simulink model "SIL_Autopilot_Vasarhelyi"  (R2020b)
settings: Solver=FixedStepAuto  StartTime=0  StopTime=T  FixedStep=0.01  RelTol=1e-3  EnableMultiTasking=on
model workspace (MAT data in the model file):
  SL_ROS_VariableLengthArrays_MaxSizes : object (value not decoded)
undefined symbols (not defined in the file): Altitude_ref, DiscIntNeverNeededParam, Elevators, p_swarm, Propeller, RightAileron, RightFlap, Rudder
libraries: robotlib x20, simulink x15
(part 2 of 5)

== system SIL_Autopilot_Vasarhelyi/Cessna 4/Attitude Control ==
  note: bota po
  Vel ref : Inport
  Euler Angles : Inport  Port=2
  Roll_ref : Inport  Port=3
  Altitude : Inport  Port=4
  Vel_in : Inport  Port=5
  Altitude ref : Inport  Port=6
  Bus Selector : BusSelector  OutputSignals=Pitch,Roll,Yaw
  Constant : Constant  Value=0
  Controle de Altitude : Subsystem
  Controle de Velocidade : Subsystem
  Gain : Gain  Gain=-1
  Servo : Subsystem
  Sum1 : Sum  Inputs=|+-
  Sum3 : Sum  Inputs=+-|
  Sum5 : Sum  Inputs=+-|
  Z Take-off Ref : Constant  Value=5
  Profundor : Outport
  Rudder : Outport  Port=2
  Aileron : Outport  Port=3
  Throtlle : Outport  Port=4
  altitude_e : Outport  Port=5
  velocity_e : Outport  Port=6
  roll_e : Outport  Port=7
  wires:
  Roll_ref/1 -> Sum1/1  "Roll Ref"
  Constant/1 -> Sum5/1  "Yaw Ref"
  Servo/4(Throtlle) -> Throtlle/1
  Servo/2(Aileron) -> Aileron/1
  Servo/3(Rudder) -> Rudder/1
  Servo/1(Profundor) -> Profundor/1
  Z Take-off Ref/1 -> Servo/6(Altitude Ref)
  Altitude/1 -> Controle de Altitude/2(Altitude), Servo/5(Altitude)
  Gain/1 -> Sum3/2
  Sum5/1 -> Servo/3(Yaw Attitude)
  Bus Selector/3 -> Sum5/2  "<Yaw>"
  Sum3/1 -> Servo/1(Pitch Attitude)
  Euler Angles/1 -> Bus Selector/1
  Bus Selector/1 -> Gain/1  "<Pitch>"
  Bus Selector/2 -> Sum1/2  "<Roll>"
  Controle de Velocidade/1(Propeller Target) -> Servo/4(Vel_in)
  Controle de Altitude/1(Pitch_ref) -> Sum3/1
  Vel ref/1 -> Controle de Velocidade/1(Velocity Ref)
  Altitude ref/1 -> Controle de Altitude/1(Altitude Ref)
  Sum1/1 -> roll_e/1, Servo/2(Roll Attitude)
  Vel_in/1 -> Controle de Velocidade/2(Velocity)
  Controle de Altitude/2(altitude_error) -> altitude_e/1
  Controle de Velocidade/2(velocity_error) -> velocity_e/1

== system SIL_Autopilot_Vasarhelyi/Cessna 4/Controle de Direção ==
  Yaw : Inport
  X : Inport  Port=2
  Y : Inport  Port=3
  Y Ref : Inport  Port=4
  X Ref : Inport  Port=5
  Atan2 : Trigonometry  Operator=atan2
  Discrete Derivative : simulink/Discrete/Discrete Derivative  gainval=1.0  ICPrevScaledInput=0.0  OutMin=[]  OutMax=[]  OutDataType=fixdt(1, 16)  OutScaling=2^-10  DoSatur=off
  Discrete-Time Integrator : DiscreteIntegrator  SampleTime=-1  ICPrevOutput=DiscIntNeverNeededParam  ICPrevScaledInput=DiscIntNeverNeededParam
  Kd : Gain  Gain=3.0
  Ki : Gain  Gain=0.0
  Kp : Gain  Gain=1.6616
  Mux1 : Mux  Inputs=2
  Mux2 : Mux  Inputs=2
  Mux3 : Mux  Inputs=2
  Saturation : Saturate  UpperLimit=0.226893  LowerLimit=-0.226893
  Sum2 : Sum  Inputs=|+-
  Sum3 : Sum  Inputs=|+-
  Sum4 : Sum  Inputs=|+-
  Sum5 : Sum  Inputs=+++
  neg : Gain  Gain=-1
  yaw_error : Outport
  Roll Ref : Outport  Port=2
  guidance_error : Outport  Port=3
  wires:
  Mux1/1 -> Mux3/1
  Mux2/1 -> Mux3/2
  Saturation/1 -> neg/1
  neg/1 -> Roll Ref/1
  Sum3/1 -> Atan2/1
  Y/1 -> Sum3/2, Mux2/2
  Y Ref/1 -> Sum3/1, Mux2/1
  X Ref/1 -> Sum2/1, Mux1/1
  X/1 -> Sum2/2, Mux1/2
  Sum2/1 -> Atan2/2
  Atan2/1 -> Sum4/1
  Yaw/1 -> Sum4/2
  Mux3/1 -> guidance_error/1
  Sum5/1 -> Saturation/1
  Kp/1 -> Sum5/2
  Kd/1 -> Sum5/1
  Discrete Derivative/1 -> Kd/1
  Discrete-Time Integrator/1 -> Ki/1
  Sum4/1 -> Discrete-Time Integrator/1, Kp/1, Discrete Derivative/1, yaw_error/1
  Ki/1 -> Sum5/3

== system SIL_Autopilot_Vasarhelyi/Cessna 4/Local Flocking Algorithm ==
  Pos : Inport
  Altitude ref : Inport  Port=2
  Xi : Inport  Port=3
  Bus Selector2 : BusSelector  OutputSignals=X,Y,Altitude
  Discrete Derivative : simulink/Discrete/Discrete Derivative  gainval=1.0  ICPrevScaledInput=0.0  OutMin=[]  OutMax=[]  OutDataType=fixdt(1, 16)  OutScaling=2^-10  DoSatur=off
  Gerador de Waypoints : Subsystem
  Mux : Mux  Inputs=3
  Mux1 : Mux  Inputs=3
  Vasarhelyi Algorithm : Subsystem
  Velocity Direction : MATLAB Function  TreatAsAtomicUnit=on
  Z : Display
  Y Ref : Outport
  X Ref : Outport  Port=2
  vel : Outport  Port=3
  u_ref : Outport  Port=4
  Waypoints : Outport  Port=5
  wires:
  Mux1/1 -> Waypoints/1, Velocity Direction/2(wp)
  Velocity Direction/1(u_ref) -> u_ref/1, Vasarhelyi Algorithm/3(u_ref)
  Pos/1 -> Bus Selector2/1
  Altitude ref/1 -> Mux1/3
  Gerador de Waypoints/2(Y Ref) -> Mux1/2
  Gerador de Waypoints/1(X Ref) -> Mux1/1
  Bus Selector2/1 -> Gerador de Waypoints/1(X State), Mux/1  "<X>"
  Bus Selector2/2 -> Gerador de Waypoints/2(Y State), Mux/2  "<Y>"
  Bus Selector2/3 -> Mux/3  "<Altitude>"
  Mux/1 -> Discrete Derivative/1, Vasarhelyi Algorithm/1(pos_i), Velocity Direction/1(pos)
  Discrete Derivative/1 -> vel/1
  Xi/1 -> Vasarhelyi Algorithm/2(pqj)
  Vasarhelyi Algorithm/1(X) -> X Ref/1
  Vasarhelyi Algorithm/2(Y) -> Y Ref/1
  Vasarhelyi Algorithm/3(Z) -> Z/1

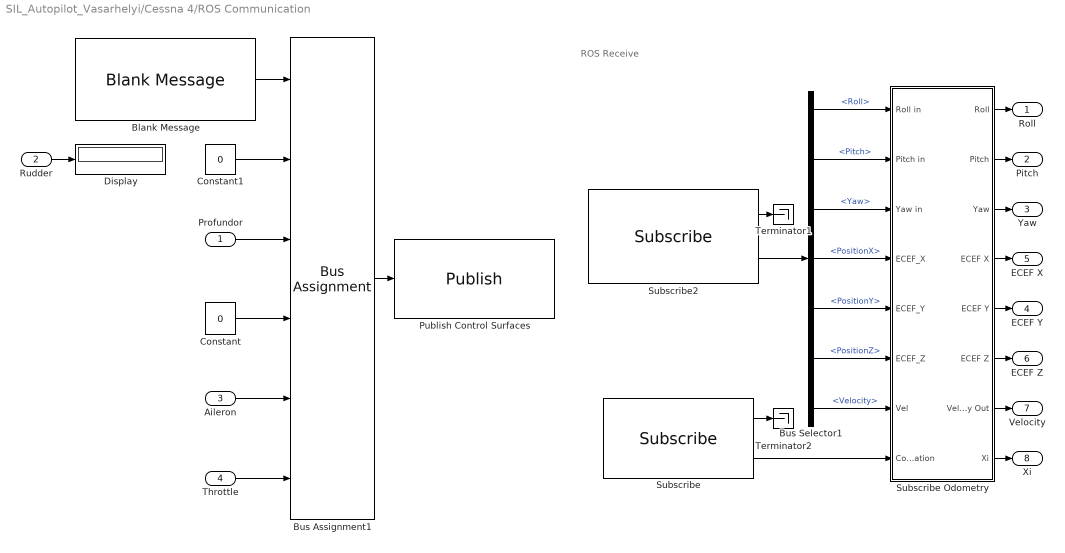
== system SIL_Autopilot_Vasarhelyi/Cessna 4/ROS Communication ==
  note: ROS Receive
  Profundor : Inport
  Rudder : Inport  Port=2
  Aileron : Inport  Port=3
  Throttle : Inport  Port=4
  Blank Message : robotlib/Blank Message  messageClass=Message  entityType=cessna_control/control_surfaces  messageType=cessna_control/control_surfaces  SampleTime=0.01  legacyBusStruct=off
  Bus Assignment1 : BusAssignment  AssignedSignals=Rudder,Elevators,RightFlap,RightAileron,Propeller
  Bus Selector1 : BusSelector  OutputSignals=Roll,Pitch,Yaw,PositionX,PositionY,PositionZ,Velocity
  Constant : Constant  Value=0
  Constant1 : Constant  Value=0
  Display : Display
  Publish Control Surfaces : robotlib/Publish  topicSource=Select from ROS network  topic=/uav4/cmd_control_surfaces  messageType=cessna_control/control_surfaces  legacyBusStruct=off  messageQueueLength=1
  Subscribe : robotlib/Subscribe  topicSource=Select from ROS network  topic=/uav4/Communication  messageType=aircraft_communication/NetworkComm  SampleTime=0.01  legacyBusStruct=off  messageQueueLength=1
  Subscribe Odometry : Subsystem  TreatAsAtomicUnit=on
  Subscribe2 : robotlib/Subscribe  topicSource=Select from ROS network  topic=/uav4/ground_truth/Odometry  messageType=aircraft_communication/Odom  SampleTime=0.01  legacyBusStruct=off  messageQueueLength=1
  Terminator1 : Terminator
  Terminator2 : Terminator
  Roll : Outport
  Pitch : Outport  Port=2
  Yaw : Outport  Port=3
  ECEF Y : Outport  Port=4
  ECEF X : Outport  Port=5
  ECEF Z : Outport  Port=6
  Velocity : Outport  Port=7
  Xi : Outport  Port=8
  wires:
  Profundor/1 -> Bus Assignment1/3
  Constant/1 -> Bus Assignment1/4
  Aileron/1 -> Bus Assignment1/5
  Subscribe Odometry/2(Pitch) -> Pitch/1
  Subscribe Odometry/4(ECEF X) -> ECEF X/1
  Subscribe Odometry/3(Yaw) -> Yaw/1
  Subscribe Odometry/1(Roll) -> Roll/1
  Subscribe Odometry/6(ECEF Z) -> ECEF Z/1
  Subscribe Odometry/7(Velocity Out) -> Velocity/1
  Rudder/1 -> Display/1
  Subscribe Odometry/8(Xi) -> Xi/1
  Throttle/1 -> Bus Assignment1/6
  Constant1/1 -> Bus Assignment1/2
  Bus Selector1/3 -> Subscribe Odometry/3(Yaw in)  "<Yaw>"
  Bus Assignment1/1 -> Publish Control Surfaces/1
  Bus Selector1/4 -> Subscribe Odometry/4(ECEF_X)  "<PositionX>"
  Bus Selector1/6 -> Subscribe Odometry/6(ECEF_Z)  "<PositionZ>"
  Blank Message/1 -> Bus Assignment1/1
  Subscribe/1 -> Terminator2/1
  Subscribe2/1 -> Terminator1/1
  Bus Selector1/2 -> Subscribe Odometry/2(Pitch in)  "<Pitch>"
  Subscribe/2 -> Subscribe Odometry/8(Communication)
  Bus Selector1/7 -> Subscribe Odometry/7(Vel)  "<Velocity>"
  Bus Selector1/1 -> Subscribe Odometry/1(Roll in)  "<Roll>"
  Bus Selector1/5 -> Subscribe Odometry/5(ECEF_Y)  "<PositionY>"
  Subscribe Odometry/5(ECEF Y) -> ECEF Y/1
  Subscribe2/2 -> Bus Selector1/1

== system SIL_Autopilot_Vasarhelyi/Cessna 5/Attitude Control ==
  note: bota po
  Vel ref : Inport
  Euler Angles : Inport  Port=2
  Roll_ref : Inport  Port=3
  Altitude : Inport  Port=4
  Vel_in : Inport  Port=5
  Altitude ref : Inport  Port=6
  Bus Selector : BusSelector  OutputSignals=Pitch,Roll,Yaw
  Constant : Constant  Value=0
  Controle de Altitude : Subsystem
  Controle de Velocidade : Subsystem
  Gain : Gain  Gain=-1
  Servo : Subsystem
  Sum1 : Sum  Inputs=|+-
  Sum3 : Sum  Inputs=+-|
  Sum5 : Sum  Inputs=+-|
  Z Take-off Ref : Constant  Value=5
  Profundor : Outport
  Rudder : Outport  Port=2
  Aileron : Outport  Port=3
  Throtlle : Outport  Port=4
  altitude_e : Outport  Port=5
  velocity_e : Outport  Port=6
  roll_e : Outport  Port=7
  wires:
  Roll_ref/1 -> Sum1/1  "Roll Ref"
  Constant/1 -> Sum5/1  "Yaw Ref"
  Servo/4(Throtlle) -> Throtlle/1
  Servo/2(Aileron) -> Aileron/1
  Servo/3(Rudder) -> Rudder/1
  Servo/1(Profundor) -> Profundor/1
  Z Take-off Ref/1 -> Servo/6(Altitude Ref)
  Altitude/1 -> Controle de Altitude/2(Altitude), Servo/5(Altitude)
  Gain/1 -> Sum3/2
  Sum5/1 -> Servo/3(Yaw Attitude)
  Bus Selector/3 -> Sum5/2  "<Yaw>"
  Sum3/1 -> Servo/1(Pitch Attitude)
  Euler Angles/1 -> Bus Selector/1
  Bus Selector/1 -> Gain/1  "<Pitch>"
  Bus Selector/2 -> Sum1/2  "<Roll>"
  Controle de Velocidade/1(Propeller Target) -> Servo/4(Vel_in)
  Controle de Altitude/1(Pitch_ref) -> Sum3/1
  Vel ref/1 -> Controle de Velocidade/1(Velocity Ref)
  Altitude ref/1 -> Controle de Altitude/1(Altitude Ref)
  Sum1/1 -> roll_e/1, Servo/2(Roll Attitude)
  Vel_in/1 -> Controle de Velocidade/2(Velocity)
  Controle de Altitude/2(altitude_error) -> altitude_e/1
  Controle de Velocidade/2(velocity_error) -> velocity_e/1

== system SIL_Autopilot_Vasarhelyi/Cessna 5/Controle de Direção ==
  Yaw : Inport
  X : Inport  Port=2
  Y : Inport  Port=3
  Y Ref : Inport  Port=4
  X Ref : Inport  Port=5
  Atan2 : Trigonometry  Operator=atan2
  Discrete Derivative : simulink/Discrete/Discrete Derivative  gainval=1.0  ICPrevScaledInput=0.0  OutMin=[]  OutMax=[]  OutDataType=fixdt(1, 16)  OutScaling=2^-10  DoSatur=off
  Discrete-Time Integrator : DiscreteIntegrator  SampleTime=-1  ICPrevOutput=DiscIntNeverNeededParam  ICPrevScaledInput=DiscIntNeverNeededParam
  Kd : Gain  Gain=3.0
  Ki : Gain  Gain=0.0
  Kp : Gain  Gain=1.6616
  Mux1 : Mux  Inputs=2
  Mux2 : Mux  Inputs=2
  Mux3 : Mux  Inputs=2
  Saturation : Saturate  UpperLimit=0.226893  LowerLimit=-0.226893
  Sum2 : Sum  Inputs=|+-
  Sum3 : Sum  Inputs=|+-
  Sum4 : Sum  Inputs=|+-
  Sum5 : Sum  Inputs=+++
  neg : Gain  Gain=-1
  yaw_error : Outport
  Roll Ref : Outport  Port=2
  guidance_error : Outport  Port=3
  wires:
  Mux1/1 -> Mux3/1
  Mux2/1 -> Mux3/2
  Saturation/1 -> neg/1
  neg/1 -> Roll Ref/1
  Sum3/1 -> Atan2/1
  Y/1 -> Sum3/2, Mux2/2
  Y Ref/1 -> Sum3/1, Mux2/1
  X Ref/1 -> Sum2/1, Mux1/1
  X/1 -> Sum2/2, Mux1/2
  Sum2/1 -> Atan2/2
  Atan2/1 -> Sum4/1
  Yaw/1 -> Sum4/2
  Mux3/1 -> guidance_error/1
  Sum5/1 -> Saturation/1
  Kp/1 -> Sum5/2
  Kd/1 -> Sum5/1
  Discrete Derivative/1 -> Kd/1
  Discrete-Time Integrator/1 -> Ki/1
  Sum4/1 -> Discrete-Time Integrator/1, Kp/1, Discrete Derivative/1, yaw_error/1
  Ki/1 -> Sum5/3

== system SIL_Autopilot_Vasarhelyi/Cessna 5/Local Flocking Algorithm ==
  Pos : Inport
  Altitude ref : Inport  Port=2
  Xi : Inport  Port=3
  Bus Selector2 : BusSelector  OutputSignals=X,Y,Altitude
  Discrete Derivative : simulink/Discrete/Discrete Derivative  gainval=1.0  ICPrevScaledInput=0.0  OutMin=[]  OutMax=[]  OutDataType=fixdt(1, 16)  OutScaling=2^-10  DoSatur=off
  Gerador de Waypoints : Subsystem
  Mux : Mux  Inputs=3
  Mux1 : Mux  Inputs=3
  Vasarhelyi Algorithm : Subsystem
  Velocity Direction : MATLAB Function  TreatAsAtomicUnit=on
  Z : Display
  Y Ref : Outport
  X Ref : Outport  Port=2
  vel : Outport  Port=3
  u_ref : Outport  Port=4
  Waypoints : Outport  Port=5
  wires:
  Mux1/1 -> Waypoints/1, Velocity Direction/2(wp)
  Velocity Direction/1(u_ref) -> u_ref/1, Vasarhelyi Algorithm/3(u_ref)
  Pos/1 -> Bus Selector2/1
  Altitude ref/1 -> Mux1/3
  Gerador de Waypoints/2(Y Ref) -> Mux1/2
  Gerador de Waypoints/1(X Ref) -> Mux1/1
  Bus Selector2/1 -> Gerador de Waypoints/1(X State), Mux/1  "<X>"
  Bus Selector2/2 -> Gerador de Waypoints/2(Y State), Mux/2  "<Y>"
  Bus Selector2/3 -> Mux/3  "<Altitude>"
  Mux/1 -> Discrete Derivative/1, Vasarhelyi Algorithm/1(pos_i), Velocity Direction/1(pos)
  Discrete Derivative/1 -> vel/1
  Xi/1 -> Vasarhelyi Algorithm/2(pqj)
  Vasarhelyi Algorithm/1(X) -> X Ref/1
  Vasarhelyi Algorithm/2(Y) -> Y Ref/1
  Vasarhelyi Algorithm/3(Z) -> Z/1

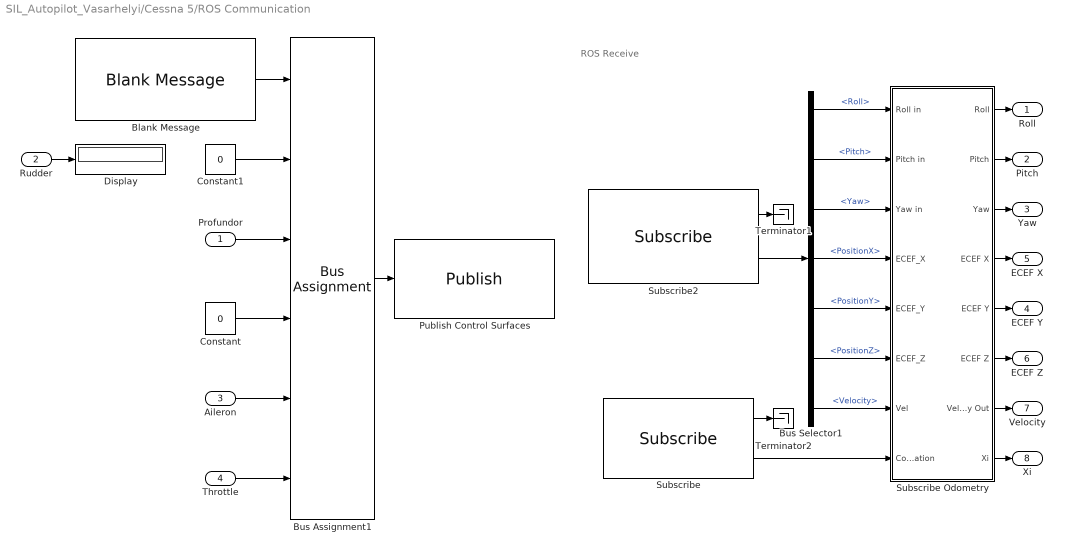
== system SIL_Autopilot_Vasarhelyi/Cessna 5/ROS Communication ==
  note: ROS Receive
  Profundor : Inport
  Rudder : Inport  Port=2
  Aileron : Inport  Port=3
  Throttle : Inport  Port=4
  Blank Message : robotlib/Blank Message  messageClass=Message  entityType=cessna_control/control_surfaces  messageType=cessna_control/control_surfaces  SampleTime=0.01  legacyBusStruct=off
  Bus Assignment1 : BusAssignment  AssignedSignals=Rudder,Elevators,RightFlap,RightAileron,Propeller
  Bus Selector1 : BusSelector  OutputSignals=Roll,Pitch,Yaw,PositionX,PositionY,PositionZ,Velocity
  Constant : Constant  Value=0
  Constant1 : Constant  Value=0
  Display : Display
  Publish Control Surfaces : robotlib/Publish  topicSource=Select from ROS network  topic=/uav5/cmd_control_surfaces  messageType=cessna_control/control_surfaces  legacyBusStruct=off  messageQueueLength=1
  Subscribe : robotlib/Subscribe  topicSource=Select from ROS network  topic=/uav5/Communication  messageType=aircraft_communication/NetworkComm  SampleTime=0.01  legacyBusStruct=off  messageQueueLength=1
  Subscribe Odometry : Subsystem  TreatAsAtomicUnit=on
  Subscribe2 : robotlib/Subscribe  topicSource=Select from ROS network  topic=/uav5/ground_truth/Odometry  messageType=aircraft_communication/Odom  SampleTime=0.01  legacyBusStruct=off  messageQueueLength=1
  Terminator1 : Terminator
  Terminator2 : Terminator
  Roll : Outport
  Pitch : Outport  Port=2
  Yaw : Outport  Port=3
  ECEF Y : Outport  Port=4
  ECEF X : Outport  Port=5
  ECEF Z : Outport  Port=6
  Velocity : Outport  Port=7
  Xi : Outport  Port=8
  wires:
  Profundor/1 -> Bus Assignment1/3
  Constant/1 -> Bus Assignment1/4
  Aileron/1 -> Bus Assignment1/5
  Subscribe Odometry/2(Pitch) -> Pitch/1
  Subscribe Odometry/4(ECEF X) -> ECEF X/1
  Subscribe Odometry/3(Yaw) -> Yaw/1
  Subscribe Odometry/1(Roll) -> Roll/1
  Subscribe Odometry/6(ECEF Z) -> ECEF Z/1
  Subscribe Odometry/7(Velocity Out) -> Velocity/1
  Rudder/1 -> Display/1
  Subscribe Odometry/8(Xi) -> Xi/1
  Throttle/1 -> Bus Assignment1/6
  Constant1/1 -> Bus Assignment1/2
  Bus Selector1/3 -> Subscribe Odometry/3(Yaw in)  "<Yaw>"
  Bus Assignment1/1 -> Publish Control Surfaces/1
  Bus Selector1/4 -> Subscribe Odometry/4(ECEF_X)  "<PositionX>"
  Bus Selector1/6 -> Subscribe Odometry/6(ECEF_Z)  "<PositionZ>"
  Blank Message/1 -> Bus Assignment1/1
  Subscribe/1 -> Terminator2/1
  Subscribe2/1 -> Terminator1/1
  Bus Selector1/2 -> Subscribe Odometry/2(Pitch in)  "<Pitch>"
  Subscribe/2 -> Subscribe Odometry/8(Communication)
  Bus Selector1/7 -> Subscribe Odometry/7(Vel)  "<Velocity>"
  Bus Selector1/1 -> Subscribe Odometry/1(Roll in)  "<Roll>"
  Bus Selector1/5 -> Subscribe Odometry/5(ECEF_Y)  "<PositionY>"
  Subscribe Odometry/5(ECEF Y) -> ECEF Y/1
  Subscribe2/2 -> Bus Selector1/1

== system SIL_Autopilot_Vasarhelyi/Cessna 1/Attitude Control/Controle de Altitude ==
  Altitude Ref : Inport
  Altitude : Inport  Port=2
  Derivative1 : Derivative
  Kd : Gain  Gain=0.00162
  Kp : Gain  Gain=0.1
  Saturation : Saturate  UpperLimit=0.785398  LowerLimit=-0.785398
  Sum : Sum  Inputs=|+-
  Sum5 : Sum  Inputs=++|
  Pitch_ref : Outport
  altitude_error : Outport  Port=2
  wires:
  Saturation/1 -> Pitch_ref/1
  Altitude Ref/1 -> Sum/1
  Altitude/1 -> Sum/2
  Kp/1 -> Sum5/2
  Kd/1 -> Sum5/1
  Derivative1/1 -> Kd/1
  Sum5/1 -> Saturation/1
  Sum/1 -> Derivative1/1, Kp/1, altitude_error/1

== system SIL_Autopilot_Vasarhelyi/Cessna 1/Attitude Control/Controle de Velocidade ==
  Velocity Ref : Inport
  Velocity : Inport  Port=2
  K_prop : Gain  Gain=0.08
  PID Velocidade : Subsystem
  Propeller Ref : Constant  Value=0.7
  Saturation3 : Saturate  UpperLimit=0.8  LowerLimit=0.6
  Sum1 : Sum  Inputs=+|+
  Sum7 : Sum  Inputs=+|-
  Target Propeller : Scope
  Velocity Error : Scope
  Propeller Target : Outport
  velocity_error : Outport  Port=2
  wires:
  Velocity/1 -> Sum7/2
  Velocity Ref/1 -> Sum7/1
  PID Velocidade/1(ev) -> K_prop/1
  Saturation3/1 -> Target Propeller/1, Propeller Target/1
  Propeller Ref/1 -> Sum1/2
  K_prop/1 -> Sum1/1
  Sum1/1 -> Saturation3/1
  Sum7/1 -> PID Velocidade/1(e_vel), velocity_error/1, Velocity Error/1

== system SIL_Autopilot_Vasarhelyi/Cessna 1/Attitude Control/Servo ==
  Pitch Attitude : Inport
  Roll Attitude : Inport  Port=2
  Yaw Attitude : Inport  Port=3
  Vel_in : Inport  Port=4
  Altitude : Inport  Port=5
  Altitude Ref : Inport  Port=6
  Gain1 : Gain  Gain=-1
  Gain2 : Gain
  Gain3 : Gain
  GreaterThanOrEqual : RelationalOperator  OutDataTypeStr=boolean  RndMeth=Simplest
  Saturation2 : Saturate  UpperLimit=0.0523599  LowerLimit=-0.0523599
  Saturation4 : Saturate  UpperLimit=0.0523599  LowerLimit=-0.0523599
  Saturation6 : Saturate  UpperLimit=0.0872665  LowerLimit=-0.0872665
  Switch{,1..3} (4 alike) : Switch  Criteria=u2 ~= 0
  Take-Off : Subsystem
  Profundor : Outport
  Aileron : Outport  Port=2
  Rudder : Outport  Port=3
  Throtlle : Outport  Port=4
  wires:
  GreaterThanOrEqual/1 -> Switch3/2, Switch2/2, Switch1/2, Switch/2
  Altitude Ref/1 -> GreaterThanOrEqual/2
  Take-Off/3(Rudder) -> Switch3/3
  Take-Off/2(Aileron) -> Switch2/3
  Altitude/1 -> GreaterThanOrEqual/1
  Switch3/1 -> Rudder/1
  Vel_in/1 -> Switch/1
  Switch/1 -> Throtlle/1
  Take-Off/4(Propeller) -> Switch/3
  Switch1/1 -> Profundor/1
  Take-Off/1(Elevators) -> Switch1/3
  Switch2/1 -> Aileron/1
  Saturation2/1 -> Switch2/1
  Saturation4/1 -> Switch1/1
  Saturation6/1 -> Switch3/1
  Gain1/1 -> Saturation6/1
  Yaw Attitude/1 -> Gain1/1
  Roll Attitude/1 -> Gain3/1
  Pitch Attitude/1 -> Gain2/1
  Gain2/1 -> Saturation4/1
  Gain3/1 -> Saturation2/1

== system SIL_Autopilot_Vasarhelyi/Cessna 1/Local Flocking Algorithm/Gerador de Waypoints ==
  X State : Inport
  Y State : Inport  Port=2
  Constant11 : Constant  Value=1000
  Constant13 : Constant  Value=-2000
  Constant14 : Constant  Value=-1000
  Constant5 : Constant  Value=-1000
  Constant6 : Constant  Value=1200
  Constant7 : Constant  Value=-1000
  Constant8 : Constant  Value=3000
  Constant9 : Constant  Value=-3000
  Demux : Demux  Outputs=8
  Display : Display
  Memory : Memory
  Próximo Waypoint : MATLAB Function  TreatAsAtomicUnit=on
  WayPoints : Mux  Inputs=8
  X Ref : Outport
  Y Ref : Outport  Port=2
  wires:
  Próximo Waypoint/2(Y_ref) -> Y Ref/1
  Próximo Waypoint/3(Estado) -> Display/1, Memory/1
  Próximo Waypoint/1(X_ref) -> X Ref/1
  Demux/1 -> Próximo Waypoint/1(wp1_X)
  Demux/2 -> Próximo Waypoint/2(wp1_Y)
  Demux/3 -> Próximo Waypoint/3(wp2_X)
  Demux/4 -> Próximo Waypoint/4(wp2_Y)
  Demux/5 -> Próximo Waypoint/5(wp3_X)
  Demux/6 -> Próximo Waypoint/6(wp3_Y)
  Demux/7 -> Próximo Waypoint/7(wp4_X)
  Demux/8 -> Próximo Waypoint/8(wp4_Y)
  WayPoints/1 -> Demux/1
  Y State/1 -> Próximo Waypoint/9(Y_med)
  X State/1 -> Próximo Waypoint/10(X_med)
  Constant7/1 -> WayPoints/2
  Constant6/1 -> WayPoints/1
  Constant9/1 -> WayPoints/4
  Constant8/1 -> WayPoints/3
  Constant5/1 -> WayPoints/5
  Constant11/1 -> WayPoints/6
  Constant14/1 -> WayPoints/8
  Constant13/1 -> WayPoints/7
  Memory/1 -> Próximo Waypoint/11("Estado ")

== system SIL_Autopilot_Vasarhelyi/Cessna 1/Local Flocking Algorithm/Vasarhelyi Algorithm ==
  pos_i : Inport
  pqj : Inport  Port=2
  u_ref : Inport  Port=3
  Agents Number : Constant  Value=5
  Demux : Demux  Outputs=3
  Discrete Derivative : simulink/Discrete/Discrete Derivative  gainval=1.0  ICPrevScaledInput=0.0  OutMin=[]  OutMax=[]  OutDataType=fixdt(1, 16)  OutScaling=2^-10  DoSatur=off
  Discrete-Time Integrator : DiscreteIntegrator  SampleTime=-1  ICPrevOutput=DiscIntNeverNeededParam  ICPrevScaledInput=DiscIntNeverNeededParam
  Parameters : Subsystem
  Vasarhelyi Algorithm : MATLAB Function  TreatAsAtomicUnit=on
  dt : Constant  Value=0.01
  pos and vel of uavs : MATLAB Function  TreatAsAtomicUnit=on
  r_agent : Constant  Value=15
  X : Outport
  Y : Outport  Port=2
  Z : Outport  Port=3
  wires:
  Agents Number/1 -> pos and vel of uavs/1(nb_agents)
  u_ref/1 -> Vasarhelyi Algorithm/4(u_ref)
  Vasarhelyi Algorithm/1(vel_command) -> Discrete-Time Integrator/1
  dt/1 -> Vasarhelyi Algorithm/5(dt)
  pqj/1 -> pos and vel of uavs/3(pqj)
  r_agent/1 -> Vasarhelyi Algorithm/6(r_agent)
  Discrete-Time Integrator/1 -> Demux/1
  pos and vel of uavs/1(pos) -> Vasarhelyi Algorithm/2(pos), Discrete Derivative/1
  Demux/2 -> Y/1
  pos_i/1 -> pos and vel of uavs/2(pos_i)
  Demux/1 -> X/1
  Demux/3 -> Z/1
  Discrete Derivative/1 -> Vasarhelyi Algorithm/3(vel)
  Parameters/1(p_swarm) -> Vasarhelyi Algorithm/1(p_swarm_par)

== system SIL_Autopilot_Vasarhelyi/Cessna 1/ROS Communication/Subscribe Odometry ==
  Roll in : Inport
  Pitch in : Inport  Port=2
  Yaw in : Inport  Port=3
  ECEF_X : Inport  Port=4
  ECEF_Y : Inport  Port=5
  ECEF_Z : Inport  Port=6
  Vel : Inport  Port=7
  Communication : Inport  Port=8
  Bus Selector3 : BusSelector  OutputSignals=Comms
  Roll : Outport
  Pitch : Outport  Port=2
  Yaw : Outport  Port=3
  ECEF X : Outport  Port=4
  ECEF Y : Outport  Port=5
  ECEF Z : Outport  Port=6
  Velocity Out : Outport  Port=7
  Xi : Outport  Port=8
  wires:
  Roll in/1 -> Roll/1
  Pitch in/1 -> Pitch/1
  Yaw in/1 -> Yaw/1
  Bus Selector3/1 -> Xi/1  "<Comms>"
  ECEF_Z/1 -> ECEF Z/1
  ECEF_Y/1 -> ECEF Y/1
  ECEF_X/1 -> ECEF X/1
  Communication/1 -> Bus Selector3/1
  Vel/1 -> Velocity Out/1

== system SIL_Autopilot_Vasarhelyi/Cessna 2/Attitude Control/Controle de Altitude ==
  Altitude Ref : Inport
  Altitude : Inport  Port=2
  Derivative1 : Derivative
  Kd : Gain  Gain=0.00162
  Kp : Gain  Gain=0.1
  Saturation : Saturate  UpperLimit=0.785398  LowerLimit=-0.785398
  Sum : Sum  Inputs=|+-
  Sum5 : Sum  Inputs=++|
  Pitch_ref : Outport
  altitude_error : Outport  Port=2
  wires:
  Saturation/1 -> Pitch_ref/1
  Altitude Ref/1 -> Sum/1
  Altitude/1 -> Sum/2
  Kp/1 -> Sum5/2
  Kd/1 -> Sum5/1
  Derivative1/1 -> Kd/1
  Sum5/1 -> Saturation/1
  Sum/1 -> Derivative1/1, Kp/1, altitude_error/1

== system SIL_Autopilot_Vasarhelyi/Cessna 2/Attitude Control/Controle de Velocidade ==
  Velocity Ref : Inport
  Velocity : Inport  Port=2
  K_prop : Gain  Gain=0.08
  PID Velocidade : Subsystem
  Propeller Ref : Constant  Value=0.7
  Saturation3 : Saturate  UpperLimit=0.8  LowerLimit=0.6
  Sum1 : Sum  Inputs=+|+
  Sum7 : Sum  Inputs=+|-
  Target Propeller : Scope
  Velocity Error : Scope
  Propeller Target : Outport
  velocity_error : Outport  Port=2
  wires:
  Velocity/1 -> Sum7/2
  Velocity Ref/1 -> Sum7/1
  PID Velocidade/1(ev) -> K_prop/1
  Saturation3/1 -> Target Propeller/1, Propeller Target/1
  Propeller Ref/1 -> Sum1/2
  K_prop/1 -> Sum1/1
  Sum1/1 -> Saturation3/1
  Sum7/1 -> PID Velocidade/1(e_vel), velocity_error/1, Velocity Error/1

== system SIL_Autopilot_Vasarhelyi/Cessna 2/Attitude Control/Servo ==
  Pitch Attitude : Inport
  Roll Attitude : Inport  Port=2
  Yaw Attitude : Inport  Port=3
  Vel_in : Inport  Port=4
  Altitude : Inport  Port=5
  Altitude Ref : Inport  Port=6
  Gain1 : Gain  Gain=-1
  Gain2 : Gain
  Gain3 : Gain
  GreaterThanOrEqual : RelationalOperator  OutDataTypeStr=boolean  RndMeth=Simplest
  Saturation2 : Saturate  UpperLimit=0.0523599  LowerLimit=-0.0523599
  Saturation4 : Saturate  UpperLimit=0.0523599  LowerLimit=-0.0523599
  Saturation6 : Saturate  UpperLimit=0.0872665  LowerLimit=-0.0872665
  Switch{,1..3} (4 alike) : Switch  Criteria=u2 ~= 0
  Take-Off : Subsystem
  Profundor : Outport
  Aileron : Outport  Port=2
  Rudder : Outport  Port=3
  Throtlle : Outport  Port=4
  wires:
  GreaterThanOrEqual/1 -> Switch3/2, Switch2/2, Switch1/2, Switch/2
  Altitude Ref/1 -> GreaterThanOrEqual/2
  Take-Off/3(Rudder) -> Switch3/3
  Take-Off/2(Aileron) -> Switch2/3
  Altitude/1 -> GreaterThanOrEqual/1
  Switch3/1 -> Rudder/1
  Vel_in/1 -> Switch/1
  Switch/1 -> Throtlle/1
  Take-Off/4(Propeller) -> Switch/3
  Switch1/1 -> Profundor/1
  Take-Off/1(Elevators) -> Switch1/3
  Switch2/1 -> Aileron/1
  Saturation2/1 -> Switch2/1
  Saturation4/1 -> Switch1/1
  Saturation6/1 -> Switch3/1
  Gain1/1 -> Saturation6/1
  Yaw Attitude/1 -> Gain1/1
  Roll Attitude/1 -> Gain3/1
  Pitch Attitude/1 -> Gain2/1
  Gain2/1 -> Saturation4/1
  Gain3/1 -> Saturation2/1

== system SIL_Autopilot_Vasarhelyi/Cessna 2/Local Flocking Algorithm/Gerador de Waypoints ==
  X State : Inport
  Y State : Inport  Port=2
  Constant11 : Constant  Value=1000
  Constant13 : Constant  Value=-2000
  Constant14 : Constant  Value=-1000
  Constant5 : Constant  Value=-1000
  Constant6 : Constant  Value=1200
  Constant7 : Constant  Value=-1000
  Constant8 : Constant  Value=3000
  Constant9 : Constant  Value=-3000
  Demux : Demux  Outputs=8
  Display : Display
  Memory : Memory
  Próximo Waypoint : MATLAB Function  TreatAsAtomicUnit=on
  WayPoints : Mux  Inputs=8
  X Ref : Outport
  Y Ref : Outport  Port=2
  wires:
  Próximo Waypoint/2(Y_ref) -> Y Ref/1
  Próximo Waypoint/3(Estado) -> Display/1, Memory/1
  Próximo Waypoint/1(X_ref) -> X Ref/1
  Demux/1 -> Próximo Waypoint/1(wp1_X)
  Demux/2 -> Próximo Waypoint/2(wp1_Y)
  Demux/3 -> Próximo Waypoint/3(wp2_X)
  Demux/4 -> Próximo Waypoint/4(wp2_Y)
  Demux/5 -> Próximo Waypoint/5(wp3_X)
  Demux/6 -> Próximo Waypoint/6(wp3_Y)
  Demux/7 -> Próximo Waypoint/7(wp4_X)
  Demux/8 -> Próximo Waypoint/8(wp4_Y)
  WayPoints/1 -> Demux/1
  Y State/1 -> Próximo Waypoint/9(Y_med)
  X State/1 -> Próximo Waypoint/10(X_med)
  Constant7/1 -> WayPoints/2
  Constant6/1 -> WayPoints/1
  Constant9/1 -> WayPoints/4
  Constant8/1 -> WayPoints/3
  Constant5/1 -> WayPoints/5
  Constant11/1 -> WayPoints/6
  Constant14/1 -> WayPoints/8
  Constant13/1 -> WayPoints/7
  Memory/1 -> Próximo Waypoint/11("Estado ")

== system SIL_Autopilot_Vasarhelyi/Cessna 2/Local Flocking Algorithm/Vasarhelyi Algorithm ==
  pos_i : Inport
  pqj : Inport  Port=2
  u_ref : Inport  Port=3
  Agents Number : Constant  Value=5
  Demux : Demux  Outputs=3
  Discrete Derivative : simulink/Discrete/Discrete Derivative  gainval=1.0  ICPrevScaledInput=0.0  OutMin=[]  OutMax=[]  OutDataType=fixdt(1, 16)  OutScaling=2^-10  DoSatur=off
  Discrete-Time Integrator : DiscreteIntegrator  SampleTime=-1  ICPrevOutput=DiscIntNeverNeededParam  ICPrevScaledInput=DiscIntNeverNeededParam
  Parameters : Subsystem
  Vasarhelyi Algorithm : MATLAB Function  TreatAsAtomicUnit=on
  dt : Constant  Value=0.01
  pos and vel of uavs : MATLAB Function  TreatAsAtomicUnit=on
  r_agent : Constant  Value=15
  X : Outport
  Y : Outport  Port=2
  Z : Outport  Port=3
  wires:
  Agents Number/1 -> pos and vel of uavs/1(nb_agents)
  u_ref/1 -> Vasarhelyi Algorithm/4(u_ref)
  Vasarhelyi Algorithm/1(vel_command) -> Discrete-Time Integrator/1
  dt/1 -> Vasarhelyi Algorithm/5(dt)
  pqj/1 -> pos and vel of uavs/3(pqj)
  r_agent/1 -> Vasarhelyi Algorithm/6(r_agent)
  Discrete-Time Integrator/1 -> Demux/1
  pos and vel of uavs/1(pos) -> Vasarhelyi Algorithm/2(pos), Discrete Derivative/1
  Demux/2 -> Y/1
  pos_i/1 -> pos and vel of uavs/2(pos_i)
  Demux/1 -> X/1
  Demux/3 -> Z/1
  Discrete Derivative/1 -> Vasarhelyi Algorithm/3(vel)
  Parameters/1(p_swarm) -> Vasarhelyi Algorithm/1(p_swarm_par)

== system SIL_Autopilot_Vasarhelyi/Cessna 2/ROS Communication/Subscribe Odometry ==
  Roll in : Inport
  Pitch in : Inport  Port=2
  Yaw in : Inport  Port=3
  ECEF_X : Inport  Port=4
  ECEF_Y : Inport  Port=5
  ECEF_Z : Inport  Port=6
  Vel : Inport  Port=7
  Communication : Inport  Port=8
  Bus Selector3 : BusSelector  OutputSignals=Comms
  Roll : Outport
  Pitch : Outport  Port=2
  Yaw : Outport  Port=3
  ECEF X : Outport  Port=4
  ECEF Y : Outport  Port=5
  ECEF Z : Outport  Port=6
  Velocity Out : Outport  Port=7
  Xi : Outport  Port=8
  wires:
  Roll in/1 -> Roll/1
  Pitch in/1 -> Pitch/1
  Yaw in/1 -> Yaw/1
  Bus Selector3/1 -> Xi/1  "<Comms>"
  ECEF_Z/1 -> ECEF Z/1
  ECEF_Y/1 -> ECEF Y/1
  ECEF_X/1 -> ECEF X/1
  Communication/1 -> Bus Selector3/1
  Vel/1 -> Velocity Out/1

== system SIL_Autopilot_Vasarhelyi/Cessna 3/Attitude Control/Controle de Altitude ==
  Altitude Ref : Inport
  Altitude : Inport  Port=2
  Derivative1 : Derivative
  Kd : Gain  Gain=0.00162
  Kp : Gain  Gain=0.1
  Saturation : Saturate  UpperLimit=0.785398  LowerLimit=-0.785398
  Sum : Sum  Inputs=|+-
  Sum5 : Sum  Inputs=++|
  Pitch_ref : Outport
  altitude_error : Outport  Port=2
  wires:
  Saturation/1 -> Pitch_ref/1
  Altitude Ref/1 -> Sum/1
  Altitude/1 -> Sum/2
  Kp/1 -> Sum5/2
  Kd/1 -> Sum5/1
  Derivative1/1 -> Kd/1
  Sum5/1 -> Saturation/1
  Sum/1 -> Derivative1/1, Kp/1, altitude_error/1

== system SIL_Autopilot_Vasarhelyi/Cessna 3/Attitude Control/Controle de Velocidade ==
  Velocity Ref : Inport
  Velocity : Inport  Port=2
  K_prop : Gain  Gain=0.08
  PID Velocidade : Subsystem
  Propeller Ref : Constant  Value=0.7
  Saturation3 : Saturate  UpperLimit=0.8  LowerLimit=0.6
  Sum1 : Sum  Inputs=+|+
  Sum7 : Sum  Inputs=+|-
  Target Propeller : Scope
  Velocity Error : Scope
  Propeller Target : Outport
  velocity_error : Outport  Port=2
  wires:
  Velocity/1 -> Sum7/2
  Velocity Ref/1 -> Sum7/1
  PID Velocidade/1(ev) -> K_prop/1
  Saturation3/1 -> Target Propeller/1, Propeller Target/1
  Propeller Ref/1 -> Sum1/2
  K_prop/1 -> Sum1/1
  Sum1/1 -> Saturation3/1
  Sum7/1 -> PID Velocidade/1(e_vel), velocity_error/1, Velocity Error/1

== system SIL_Autopilot_Vasarhelyi/Cessna 3/Attitude Control/Servo ==
  Pitch Attitude : Inport
  Roll Attitude : Inport  Port=2
  Yaw Attitude : Inport  Port=3
  Vel_in : Inport  Port=4
  Altitude : Inport  Port=5
  Altitude Ref : Inport  Port=6
  Gain1 : Gain  Gain=-1
  Gain2 : Gain
  Gain3 : Gain
  GreaterThanOrEqual : RelationalOperator  OutDataTypeStr=boolean  RndMeth=Simplest
  Saturation2 : Saturate  UpperLimit=0.0523599  LowerLimit=-0.0523599
  Saturation4 : Saturate  UpperLimit=0.0523599  LowerLimit=-0.0523599
  Saturation6 : Saturate  UpperLimit=0.0872665  LowerLimit=-0.0872665
  Switch{,1..3} (4 alike) : Switch  Criteria=u2 ~= 0
  Take-Off : Subsystem
  Profundor : Outport
  Aileron : Outport  Port=2
  Rudder : Outport  Port=3
  Throtlle : Outport  Port=4
  wires:
  GreaterThanOrEqual/1 -> Switch3/2, Switch2/2, Switch1/2, Switch/2
  Altitude Ref/1 -> GreaterThanOrEqual/2
  Take-Off/3(Rudder) -> Switch3/3
  Take-Off/2(Aileron) -> Switch2/3
  Altitude/1 -> GreaterThanOrEqual/1
  Switch3/1 -> Rudder/1
  Vel_in/1 -> Switch/1
  Switch/1 -> Throtlle/1
  Take-Off/4(Propeller) -> Switch/3
  Switch1/1 -> Profundor/1
  Take-Off/1(Elevators) -> Switch1/3
  Switch2/1 -> Aileron/1
  Saturation2/1 -> Switch2/1
  Saturation4/1 -> Switch1/1
  Saturation6/1 -> Switch3/1
  Gain1/1 -> Saturation6/1
  Yaw Attitude/1 -> Gain1/1
  Roll Attitude/1 -> Gain3/1
  Pitch Attitude/1 -> Gain2/1
  Gain2/1 -> Saturation4/1
  Gain3/1 -> Saturation2/1

== system SIL_Autopilot_Vasarhelyi/Cessna 3/Local Flocking Algorithm/Gerador de Waypoints ==
  X State : Inport
  Y State : Inport  Port=2
  Constant11 : Constant  Value=1000
  Constant13 : Constant  Value=-2000
  Constant14 : Constant  Value=-1000
  Constant5 : Constant  Value=-1000
  Constant6 : Constant  Value=1200
  Constant7 : Constant  Value=-1000
  Constant8 : Constant  Value=3000
  Constant9 : Constant  Value=-3000
  Demux : Demux  Outputs=8
  Display : Display
  Memory : Memory
  Próximo Waypoint : MATLAB Function  TreatAsAtomicUnit=on
  WayPoints : Mux  Inputs=8
  X Ref : Outport
  Y Ref : Outport  Port=2
  wires:
  Próximo Waypoint/2(Y_ref) -> Y Ref/1
  Próximo Waypoint/3(Estado) -> Display/1, Memory/1
  Próximo Waypoint/1(X_ref) -> X Ref/1
  Demux/1 -> Próximo Waypoint/1(wp1_X)
  Demux/2 -> Próximo Waypoint/2(wp1_Y)
  Demux/3 -> Próximo Waypoint/3(wp2_X)
  Demux/4 -> Próximo Waypoint/4(wp2_Y)
  Demux/5 -> Próximo Waypoint/5(wp3_X)
  Demux/6 -> Próximo Waypoint/6(wp3_Y)
  Demux/7 -> Próximo Waypoint/7(wp4_X)
  Demux/8 -> Próximo Waypoint/8(wp4_Y)
  WayPoints/1 -> Demux/1
  Y State/1 -> Próximo Waypoint/9(Y_med)
  X State/1 -> Próximo Waypoint/10(X_med)
  Constant7/1 -> WayPoints/2
  Constant6/1 -> WayPoints/1
  Constant9/1 -> WayPoints/4
  Constant8/1 -> WayPoints/3
  Constant5/1 -> WayPoints/5
  Constant11/1 -> WayPoints/6
  Constant14/1 -> WayPoints/8
  Constant13/1 -> WayPoints/7
  Memory/1 -> Próximo Waypoint/11("Estado ")

== system SIL_Autopilot_Vasarhelyi/Cessna 3/Local Flocking Algorithm/Vasarhelyi Algorithm ==
  pos_i : Inport
  pqj : Inport  Port=2
  u_ref : Inport  Port=3
  Agents Number : Constant  Value=5
  Demux : Demux  Outputs=3
  Discrete Derivative : simulink/Discrete/Discrete Derivative  gainval=1.0  ICPrevScaledInput=0.0  OutMin=[]  OutMax=[]  OutDataType=fixdt(1, 16)  OutScaling=2^-10  DoSatur=off
  Discrete-Time Integrator : DiscreteIntegrator  SampleTime=-1  ICPrevOutput=DiscIntNeverNeededParam  ICPrevScaledInput=DiscIntNeverNeededParam
  Parameters : Subsystem
  Vasarhelyi Algorithm : MATLAB Function  TreatAsAtomicUnit=on
  dt : Constant  Value=0.01
  pos and vel of uavs : MATLAB Function  TreatAsAtomicUnit=on
  r_agent : Constant  Value=15
  X : Outport
  Y : Outport  Port=2
  Z : Outport  Port=3
  wires:
  Agents Number/1 -> pos and vel of uavs/1(nb_agents)
  u_ref/1 -> Vasarhelyi Algorithm/4(u_ref)
  Vasarhelyi Algorithm/1(vel_command) -> Discrete-Time Integrator/1
  dt/1 -> Vasarhelyi Algorithm/5(dt)
  pqj/1 -> pos and vel of uavs/3(pqj)
  r_agent/1 -> Vasarhelyi Algorithm/6(r_agent)
  Discrete-Time Integrator/1 -> Demux/1
  pos and vel of uavs/1(pos) -> Vasarhelyi Algorithm/2(pos), Discrete Derivative/1
  Demux/2 -> Y/1
  pos_i/1 -> pos and vel of uavs/2(pos_i)
  Demux/1 -> X/1
  Demux/3 -> Z/1
  Discrete Derivative/1 -> Vasarhelyi Algorithm/3(vel)
  Parameters/1(p_swarm) -> Vasarhelyi Algorithm/1(p_swarm_par)

== system SIL_Autopilot_Vasarhelyi/Cessna 3/ROS Communication/Subscribe Odometry ==
  Roll in : Inport
  Pitch in : Inport  Port=2
  Yaw in : Inport  Port=3
  ECEF_X : Inport  Port=4
  ECEF_Y : Inport  Port=5
  ECEF_Z : Inport  Port=6
  Vel : Inport  Port=7
  Communication : Inport  Port=8
  Bus Selector3 : BusSelector  OutputSignals=Comms
  Roll : Outport
  Pitch : Outport  Port=2
  Yaw : Outport  Port=3
  ECEF X : Outport  Port=4
  ECEF Y : Outport  Port=5
  ECEF Z : Outport  Port=6
  Velocity Out : Outport  Port=7
  Xi : Outport  Port=8
  wires:
  Roll in/1 -> Roll/1
  Pitch in/1 -> Pitch/1
  Yaw in/1 -> Yaw/1
  Bus Selector3/1 -> Xi/1  "<Comms>"
  ECEF_Z/1 -> ECEF Z/1
  ECEF_Y/1 -> ECEF Y/1
  ECEF_X/1 -> ECEF X/1
  Communication/1 -> Bus Selector3/1
  Vel/1 -> Velocity Out/1

== system SIL_Autopilot_Vasarhelyi/Cessna 4/Attitude Control/Controle de Altitude ==
  Altitude Ref : Inport
  Altitude : Inport  Port=2
  Derivative1 : Derivative
  Kd : Gain  Gain=0.00162
  Kp : Gain  Gain=0.1
  Saturation : Saturate  UpperLimit=0.785398  LowerLimit=-0.785398
  Sum : Sum  Inputs=|+-
  Sum5 : Sum  Inputs=++|
  Pitch_ref : Outport
  altitude_error : Outport  Port=2
  wires:
  Saturation/1 -> Pitch_ref/1
  Altitude Ref/1 -> Sum/1
  Altitude/1 -> Sum/2
  Kp/1 -> Sum5/2
  Kd/1 -> Sum5/1
  Derivative1/1 -> Kd/1
  Sum5/1 -> Saturation/1
  Sum/1 -> Derivative1/1, Kp/1, altitude_error/1

== system SIL_Autopilot_Vasarhelyi/Cessna 4/Attitude Control/Controle de Velocidade ==
  Velocity Ref : Inport
  Velocity : Inport  Port=2
  K_prop : Gain  Gain=0.08
  PID Velocidade : Subsystem
  Propeller Ref : Constant  Value=0.7
  Saturation3 : Saturate  UpperLimit=0.8  LowerLimit=0.6
  Sum1 : Sum  Inputs=+|+
  Sum7 : Sum  Inputs=+|-
  Target Propeller : Scope
  Velocity Error : Scope
  Propeller Target : Outport
  velocity_error : Outport  Port=2
  wires:
  Velocity/1 -> Sum7/2
  Velocity Ref/1 -> Sum7/1
  PID Velocidade/1(ev) -> K_prop/1
  Saturation3/1 -> Target Propeller/1, Propeller Target/1
  Propeller Ref/1 -> Sum1/2
  K_prop/1 -> Sum1/1
  Sum1/1 -> Saturation3/1
  Sum7/1 -> PID Velocidade/1(e_vel), velocity_error/1, Velocity Error/1

== system SIL_Autopilot_Vasarhelyi/Cessna 4/Attitude Control/Servo ==
  Pitch Attitude : Inport
  Roll Attitude : Inport  Port=2
  Yaw Attitude : Inport  Port=3
  Vel_in : Inport  Port=4
  Altitude : Inport  Port=5
  Altitude Ref : Inport  Port=6
  Gain1 : Gain  Gain=-1
  Gain2 : Gain
  Gain3 : Gain
  GreaterThanOrEqual : RelationalOperator  OutDataTypeStr=boolean  RndMeth=Simplest
  Saturation2 : Saturate  UpperLimit=0.0523599  LowerLimit=-0.0523599
  Saturation4 : Saturate  UpperLimit=0.0523599  LowerLimit=-0.0523599
  Saturation6 : Saturate  UpperLimit=0.0872665  LowerLimit=-0.0872665
  Switch{,1..3} (4 alike) : Switch  Criteria=u2 ~= 0
  Take-Off : Subsystem
  Profundor : Outport
  Aileron : Outport  Port=2
  Rudder : Outport  Port=3
  Throtlle : Outport  Port=4
  wires:
  GreaterThanOrEqual/1 -> Switch3/2, Switch2/2, Switch1/2, Switch/2
  Altitude Ref/1 -> GreaterThanOrEqual/2
  Take-Off/3(Rudder) -> Switch3/3
  Take-Off/2(Aileron) -> Switch2/3
  Altitude/1 -> GreaterThanOrEqual/1
  Switch3/1 -> Rudder/1
  Vel_in/1 -> Switch/1
  Switch/1 -> Throtlle/1
  Take-Off/4(Propeller) -> Switch/3
  Switch1/1 -> Profundor/1
  Take-Off/1(Elevators) -> Switch1/3
  Switch2/1 -> Aileron/1
  Saturation2/1 -> Switch2/1
  Saturation4/1 -> Switch1/1
  Saturation6/1 -> Switch3/1
  Gain1/1 -> Saturation6/1
  Yaw Attitude/1 -> Gain1/1
  Roll Attitude/1 -> Gain3/1
  Pitch Attitude/1 -> Gain2/1
  Gain2/1 -> Saturation4/1
  Gain3/1 -> Saturation2/1

== system SIL_Autopilot_Vasarhelyi/Cessna 4/Local Flocking Algorithm/Gerador de Waypoints ==
  X State : Inport
  Y State : Inport  Port=2
  Constant11 : Constant  Value=1000
  Constant13 : Constant  Value=-2000
  Constant14 : Constant  Value=-1000
  Constant5 : Constant  Value=-1000
  Constant6 : Constant  Value=1200
  Constant7 : Constant  Value=-1000
  Constant8 : Constant  Value=3000
  Constant9 : Constant  Value=-3000
  Demux : Demux  Outputs=8
  Display : Display
  Memory : Memory
  Próximo Waypoint : MATLAB Function  TreatAsAtomicUnit=on
  WayPoints : Mux  Inputs=8
  X Ref : Outport
  Y Ref : Outport  Port=2
  wires:
  Próximo Waypoint/2(Y_ref) -> Y Ref/1
  Próximo Waypoint/3(Estado) -> Display/1, Memory/1
  Próximo Waypoint/1(X_ref) -> X Ref/1
  Demux/1 -> Próximo Waypoint/1(wp1_X)
  Demux/2 -> Próximo Waypoint/2(wp1_Y)
  Demux/3 -> Próximo Waypoint/3(wp2_X)
  Demux/4 -> Próximo Waypoint/4(wp2_Y)
  Demux/5 -> Próximo Waypoint/5(wp3_X)
  Demux/6 -> Próximo Waypoint/6(wp3_Y)
  Demux/7 -> Próximo Waypoint/7(wp4_X)
  Demux/8 -> Próximo Waypoint/8(wp4_Y)
  WayPoints/1 -> Demux/1
  Y State/1 -> Próximo Waypoint/9(Y_med)
  X State/1 -> Próximo Waypoint/10(X_med)
  Constant7/1 -> WayPoints/2
  Constant6/1 -> WayPoints/1
  Constant9/1 -> WayPoints/4
  Constant8/1 -> WayPoints/3
  Constant5/1 -> WayPoints/5
  Constant11/1 -> WayPoints/6
  Constant14/1 -> WayPoints/8
  Constant13/1 -> WayPoints/7
  Memory/1 -> Próximo Waypoint/11("Estado ")

== system SIL_Autopilot_Vasarhelyi/Cessna 4/Local Flocking Algorithm/Vasarhelyi Algorithm ==
  pos_i : Inport
  pqj : Inport  Port=2
  u_ref : Inport  Port=3
  Agents Number : Constant  Value=5
  Demux : Demux  Outputs=3
  Discrete Derivative : simulink/Discrete/Discrete Derivative  gainval=1.0  ICPrevScaledInput=0.0  OutMin=[]  OutMax=[]  OutDataType=fixdt(1, 16)  OutScaling=2^-10  DoSatur=off
  Discrete-Time Integrator : DiscreteIntegrator  SampleTime=-1  ICPrevOutput=DiscIntNeverNeededParam  ICPrevScaledInput=DiscIntNeverNeededParam
  Parameters : Subsystem
  Vasarhelyi Algorithm : MATLAB Function  TreatAsAtomicUnit=on
  dt : Constant  Value=0.01
  pos and vel of uavs : MATLAB Function  TreatAsAtomicUnit=on
  r_agent : Constant  Value=15
  X : Outport
  Y : Outport  Port=2
  Z : Outport  Port=3
  wires:
  Agents Number/1 -> pos and vel of uavs/1(nb_agents)
  u_ref/1 -> Vasarhelyi Algorithm/4(u_ref)
  Vasarhelyi Algorithm/1(vel_command) -> Discrete-Time Integrator/1
  dt/1 -> Vasarhelyi Algorithm/5(dt)
  pqj/1 -> pos and vel of uavs/3(pqj)
  r_agent/1 -> Vasarhelyi Algorithm/6(r_agent)
  Discrete-Time Integrator/1 -> Demux/1
  pos and vel of uavs/1(pos) -> Vasarhelyi Algorithm/2(pos), Discrete Derivative/1
  Demux/2 -> Y/1
  pos_i/1 -> pos and vel of uavs/2(pos_i)
  Demux/1 -> X/1
  Demux/3 -> Z/1
  Discrete Derivative/1 -> Vasarhelyi Algorithm/3(vel)
  Parameters/1(p_swarm) -> Vasarhelyi Algorithm/1(p_swarm_par)

== system SIL_Autopilot_Vasarhelyi/Cessna 4/ROS Communication/Subscribe Odometry ==
  Roll in : Inport
  Pitch in : Inport  Port=2
  Yaw in : Inport  Port=3
  ECEF_X : Inport  Port=4
  ECEF_Y : Inport  Port=5
  ECEF_Z : Inport  Port=6
  Vel : Inport  Port=7
  Communication : Inport  Port=8
  Bus Selector3 : BusSelector  OutputSignals=Comms
  Roll : Outport
  Pitch : Outport  Port=2
  Yaw : Outport  Port=3
  ECEF X : Outport  Port=4
  ECEF Y : Outport  Port=5
  ECEF Z : Outport  Port=6
  Velocity Out : Outport  Port=7
  Xi : Outport  Port=8
  wires:
  Roll in/1 -> Roll/1
  Pitch in/1 -> Pitch/1
  Yaw in/1 -> Yaw/1
  Bus Selector3/1 -> Xi/1  "<Comms>"
  ECEF_Z/1 -> ECEF Z/1
  ECEF_Y/1 -> ECEF Y/1
  ECEF_X/1 -> ECEF X/1
  Communication/1 -> Bus Selector3/1
  Vel/1 -> Velocity Out/1

== system SIL_Autopilot_Vasarhelyi/Cessna 5/Attitude Control/Controle de Altitude ==
  Altitude Ref : Inport
  Altitude : Inport  Port=2
  Derivative1 : Derivative
  Kd : Gain  Gain=0.00162
  Kp : Gain  Gain=0.1
  Saturation : Saturate  UpperLimit=0.785398  LowerLimit=-0.785398
  Sum : Sum  Inputs=|+-
  Sum5 : Sum  Inputs=++|
  Pitch_ref : Outport
  altitude_error : Outport  Port=2
  wires:
  Saturation/1 -> Pitch_ref/1
  Altitude Ref/1 -> Sum/1
  Altitude/1 -> Sum/2
  Kp/1 -> Sum5/2
  Kd/1 -> Sum5/1
  Derivative1/1 -> Kd/1
  Sum5/1 -> Saturation/1
  Sum/1 -> Derivative1/1, Kp/1, altitude_error/1

== system SIL_Autopilot_Vasarhelyi/Cessna 5/Attitude Control/Controle de Velocidade ==
  Velocity Ref : Inport
  Velocity : Inport  Port=2
  K_prop : Gain  Gain=0.08
  PID Velocidade : Subsystem
  Propeller Ref : Constant  Value=0.7
  Saturation3 : Saturate  UpperLimit=0.8  LowerLimit=0.6
  Sum1 : Sum  Inputs=+|+
  Sum7 : Sum  Inputs=+|-
  Target Propeller : Scope
  Velocity Error : Scope
  Propeller Target : Outport
  velocity_error : Outport  Port=2
  wires:
  Velocity/1 -> Sum7/2
  Velocity Ref/1 -> Sum7/1
  PID Velocidade/1(ev) -> K_prop/1
  Saturation3/1 -> Target Propeller/1, Propeller Target/1
  Propeller Ref/1 -> Sum1/2
  K_prop/1 -> Sum1/1
  Sum1/1 -> Saturation3/1
  Sum7/1 -> PID Velocidade/1(e_vel), velocity_error/1, Velocity Error/1

== system SIL_Autopilot_Vasarhelyi/Cessna 5/Attitude Control/Servo ==
  Pitch Attitude : Inport
  Roll Attitude : Inport  Port=2
  Yaw Attitude : Inport  Port=3
  Vel_in : Inport  Port=4
  Altitude : Inport  Port=5
  Altitude Ref : Inport  Port=6
  Gain1 : Gain  Gain=-1
  Gain2 : Gain
  Gain3 : Gain
  GreaterThanOrEqual : RelationalOperator  OutDataTypeStr=boolean  RndMeth=Simplest
  Saturation2 : Saturate  UpperLimit=0.0523599  LowerLimit=-0.0523599
  Saturation4 : Saturate  UpperLimit=0.0523599  LowerLimit=-0.0523599
  Saturation6 : Saturate  UpperLimit=0.0872665  LowerLimit=-0.0872665
  Switch{,1..3} (4 alike) : Switch  Criteria=u2 ~= 0
  Take-Off : Subsystem
  Profundor : Outport
  Aileron : Outport  Port=2
  Rudder : Outport  Port=3
  Throtlle : Outport  Port=4
  wires:
  GreaterThanOrEqual/1 -> Switch3/2, Switch2/2, Switch1/2, Switch/2
  Altitude Ref/1 -> GreaterThanOrEqual/2
  Take-Off/3(Rudder) -> Switch3/3
  Take-Off/2(Aileron) -> Switch2/3
  Altitude/1 -> GreaterThanOrEqual/1
  Switch3/1 -> Rudder/1
  Vel_in/1 -> Switch/1
  Switch/1 -> Throtlle/1
  Take-Off/4(Propeller) -> Switch/3
  Switch1/1 -> Profundor/1
  Take-Off/1(Elevators) -> Switch1/3
  Switch2/1 -> Aileron/1
  Saturation2/1 -> Switch2/1
  Saturation4/1 -> Switch1/1
  Saturation6/1 -> Switch3/1
  Gain1/1 -> Saturation6/1
  Yaw Attitude/1 -> Gain1/1
  Roll Attitude/1 -> Gain3/1
  Pitch Attitude/1 -> Gain2/1
  Gain2/1 -> Saturation4/1
  Gain3/1 -> Saturation2/1

== system SIL_Autopilot_Vasarhelyi/Cessna 5/Local Flocking Algorithm/Gerador de Waypoints ==
  X State : Inport
  Y State : Inport  Port=2
  Constant11 : Constant  Value=1000
  Constant13 : Constant  Value=-2000
  Constant14 : Constant  Value=-1000
  Constant5 : Constant  Value=-1000
  Constant6 : Constant  Value=1200
  Constant7 : Constant  Value=-1000
  Constant8 : Constant  Value=3000
  Constant9 : Constant  Value=-3000
  Demux : Demux  Outputs=8
  Display : Display
  Memory : Memory
  Próximo Waypoint : MATLAB Function  TreatAsAtomicUnit=on
  WayPoints : Mux  Inputs=8
  X Ref : Outport
  Y Ref : Outport  Port=2
  wires:
  Próximo Waypoint/2(Y_ref) -> Y Ref/1
  Próximo Waypoint/3(Estado) -> Display/1, Memory/1
  Próximo Waypoint/1(X_ref) -> X Ref/1
  Demux/1 -> Próximo Waypoint/1(wp1_X)
  Demux/2 -> Próximo Waypoint/2(wp1_Y)
  Demux/3 -> Próximo Waypoint/3(wp2_X)
  Demux/4 -> Próximo Waypoint/4(wp2_Y)
  Demux/5 -> Próximo Waypoint/5(wp3_X)
  Demux/6 -> Próximo Waypoint/6(wp3_Y)
  Demux/7 -> Próximo Waypoint/7(wp4_X)
  Demux/8 -> Próximo Waypoint/8(wp4_Y)
  WayPoints/1 -> Demux/1
  Y State/1 -> Próximo Waypoint/9(Y_med)
  X State/1 -> Próximo Waypoint/10(X_med)
  Constant7/1 -> WayPoints/2
  Constant6/1 -> WayPoints/1
  Constant9/1 -> WayPoints/4
  Constant8/1 -> WayPoints/3
  Constant5/1 -> WayPoints/5
  Constant11/1 -> WayPoints/6
  Constant14/1 -> WayPoints/8
  Constant13/1 -> WayPoints/7
  Memory/1 -> Próximo Waypoint/11("Estado ")

== system SIL_Autopilot_Vasarhelyi/Cessna 5/Local Flocking Algorithm/Vasarhelyi Algorithm ==
  pos_i : Inport
  pqj : Inport  Port=2
  u_ref : Inport  Port=3
  Agents Number : Constant  Value=5
  Demux : Demux  Outputs=3
  Discrete Derivative : simulink/Discrete/Discrete Derivative  gainval=1.0  ICPrevScaledInput=0.0  OutMin=[]  OutMax=[]  OutDataType=fixdt(1, 16)  OutScaling=2^-10  DoSatur=off
  Discrete-Time Integrator : DiscreteIntegrator  SampleTime=-1  ICPrevOutput=DiscIntNeverNeededParam  ICPrevScaledInput=DiscIntNeverNeededParam
  Parameters : Subsystem
  Vasarhelyi Algorithm : MATLAB Function  TreatAsAtomicUnit=on
  dt : Constant  Value=0.01
  pos and vel of uavs : MATLAB Function  TreatAsAtomicUnit=on
  r_agent : Constant  Value=15
  X : Outport
  Y : Outport  Port=2
  Z : Outport  Port=3
  wires:
  Agents Number/1 -> pos and vel of uavs/1(nb_agents)
  u_ref/1 -> Vasarhelyi Algorithm/4(u_ref)
  Vasarhelyi Algorithm/1(vel_command) -> Discrete-Time Integrator/1
  dt/1 -> Vasarhelyi Algorithm/5(dt)
  pqj/1 -> pos and vel of uavs/3(pqj)
  r_agent/1 -> Vasarhelyi Algorithm/6(r_agent)
  Discrete-Time Integrator/1 -> Demux/1
  pos and vel of uavs/1(pos) -> Vasarhelyi Algorithm/2(pos), Discrete Derivative/1
  Demux/2 -> Y/1
  pos_i/1 -> pos and vel of uavs/2(pos_i)
  Demux/1 -> X/1
  Demux/3 -> Z/1
  Discrete Derivative/1 -> Vasarhelyi Algorithm/3(vel)
  Parameters/1(p_swarm) -> Vasarhelyi Algorithm/1(p_swarm_par)

== system SIL_Autopilot_Vasarhelyi/Cessna 5/ROS Communication/Subscribe Odometry ==
  Roll in : Inport
  Pitch in : Inport  Port=2
  Yaw in : Inport  Port=3
  ECEF_X : Inport  Port=4
  ECEF_Y : Inport  Port=5
  ECEF_Z : Inport  Port=6
  Vel : Inport  Port=7
  Communication : Inport  Port=8
  Bus Selector3 : BusSelector  OutputSignals=Comms
  Roll : Outport
  Pitch : Outport  Port=2
  Yaw : Outport  Port=3
  ECEF X : Outport  Port=4
  ECEF Y : Outport  Port=5
  ECEF Z : Outport  Port=6
  Velocity Out : Outport  Port=7
  Xi : Outport  Port=8
  wires:
  Roll in/1 -> Roll/1
  Pitch in/1 -> Pitch/1
  Yaw in/1 -> Yaw/1
  Bus Selector3/1 -> Xi/1  "<Comms>"
  ECEF_Z/1 -> ECEF Z/1
  ECEF_Y/1 -> ECEF Y/1
  ECEF_X/1 -> ECEF X/1
  Communication/1 -> Bus Selector3/1
  Vel/1 -> Velocity Out/1

== system SIL_Autopilot_Vasarhelyi/Cessna 1/Attitude Control/Controle de Velocidade/PID Velocidade ==
  e_vel : Inport
  Derivative : Derivative
  Discrete-Time Integrator : DiscreteIntegrator  SampleTime=-1  ICPrevOutput=DiscIntNeverNeededParam  ICPrevScaledInput=DiscIntNeverNeededParam
  Kd : Gain  Gain=0.05
  Ki : Gain  Gain=0.00
  Kp : Gain  Gain=0.05
  Sum2 : Sum  Inputs=+++
  ev : Outport
  wires:
  e_vel/1 -> Discrete-Time Integrator/1, Derivative/1, Kp/1
  Sum2/1 -> ev/1
  Kp/1 -> Sum2/1
  Discrete-Time Integrator/1 -> Ki/1
  Kd/1 -> Sum2/3
  Ki/1 -> Sum2/2
  Derivative/1 -> Kd/1

== system SIL_Autopilot_Vasarhelyi/Cessna 1/Attitude Control/Servo/Take-Off ==
  Constant : Constant  Value=-0.035
  Constant1 : Constant  Value=0.0436332
  Constant2 : Constant  Value=0.017
  Constant3 : Constant  Value=0.8
  Elevators : Outport
  Aileron : Outport  Port=2
  Rudder : Outport  Port=3
  Propeller : Outport  Port=4
  wires:
  Constant/1 -> Rudder/1
  Constant2/1 -> Aileron/1
  Constant3/1 -> Propeller/1
  Constant1/1 -> Elevators/1
